simulink model "PC_Quadcopter_Simulation_Hexacopter_health_wind"  (R2022b)
settings: Solver=ode4  StartTime=0.0  StopTime=100  FixedStep=0.01  MaxStep=0.06  RelTol=1e-3
PreLoadFcn:
  | DoB_parameter
model workspace (MAT data in the model file):
  Sig : Simulink.Signal (value not decoded)
values from neighbouring files (symbols this model uses):
  A = [ ... (first row only)    [DoB_parameter.m]
  B = [0 1 0]'    [DoB_parameter.m]
  C = [1 0 0]    [DoB_parameter.m]
  den_Inv_X = conv(num_X,den_Qfilter)    [DoB_parameter.m]
  den_Inv_Y = conv(num_Y, den_Qfilter)    [DoB_parameter.m]
  den_Inv_Z = conv(num_Z, den_Qfilter_Z)    [DoB_parameter.m]
  den_Qfilter = [1 a1/tau a0/tau^2]    [DoB_parameter.m]
  den_Qfilter_Z = [1 a1/tau a0/tau^2]    [DoB_parameter.m]
  I_xx = J(1,1)    [DoB_parameter.m]
  I_yy = J(2,2)    [DoB_parameter.m]
  I_zz = J(3,3)    [DoB_parameter.m]
  IC = block.DialogPrm(2).Data    [quadcopterDynamicsSFunction.m]
  L = [l1 l2 l3]'    [DoB_parameter.m]
  num_Inv_X = conv(den_X,num_Qfilter)    [DoB_parameter.m]
  num_Inv_Y = conv(den_Y, num_Qfilter)    [DoB_parameter.m]
  num_Inv_Z = conv(den_Z, num_Qfilter_Z)    [DoB_parameter.m]
  num_Qfilter = a0/tau^2    (= 100)    [DoB_parameter.m]
  num_Qfilter_Z = a0/tau^2    (= 11.1111111111)    [DoB_parameter.m]
undefined symbols (not defined in the file or in its folder): F, Light, magnitude, MIL, quadModel
libraries: simulink x37, sharedTrackingLibrary x1, aerolibwind2 x1
(part 2 of 3)

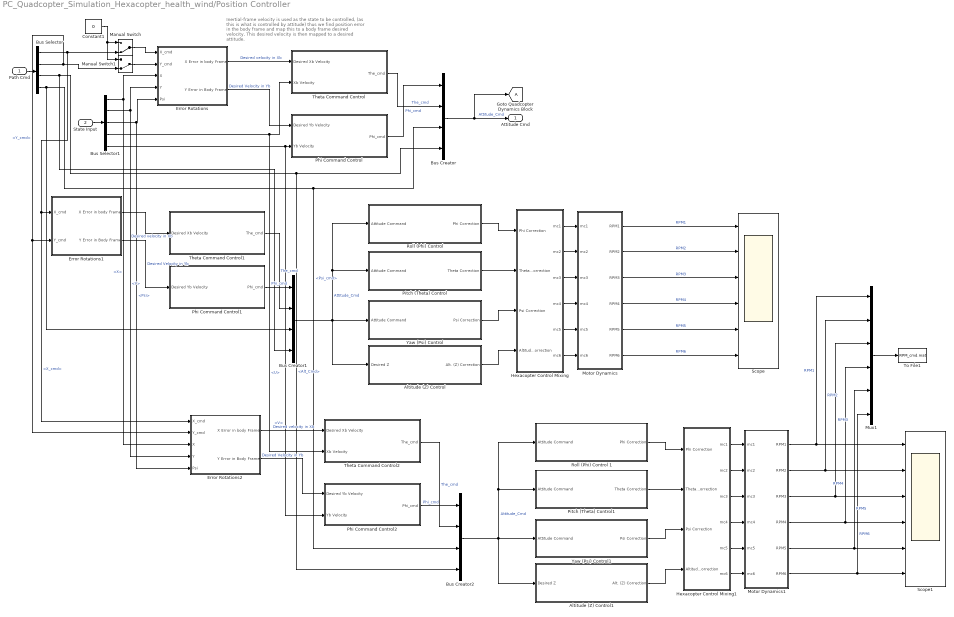
== system PC_Quadcopter_Simulation_Hexacopter_health_wind/Position Controller ==
  note: Inertial-frame velocity is used as the state to be controlled,
      | (as this is what is controlled by attitude)
      | thus we find position error in the body frame
      | and map this to a body frame desired velocity. This desired
      | velocity is then mapped to a desired attitude.
  Path Cmd : Inport
  State Input : Inport  Port=2
  Altitude (Z) Control : Subsystem  mask{Kpz=9, Kiz=6.6, Kdz=9.9, LimitOutput=on, USat=1, LSat=-1, GOffset=(sqrt((quadModel.mass*quadModel.g)/(6*quadModel.ct))-quadModel.b)/quadModel.cr}
      mask prompts: Kpz "Kp"; Kiz "Ki"; Kdz "Kd"; LimitOutput "Integral Saturation?"; USat "Upper saturation limit:"; LSat "Lower saturation limit:"; GOffset "Gravity Feedforward"
      mask help:
      | Adjust PID controller gains through this mask interface, or "look under mask" for more detailed adjustments.
      |
      | Note: Gravity Offset will not appear on block face as a value until simulation is run if it is the result of a formula involving the quadcopter model parameters.
      mask TypeOptions Kpz: Kpz/Gain
      mask TypeOptions Kiz: Kiz/Gain
      mask TypeOptions Kdz: Kdz/Gain
      mask TypeOptions LimitOutput:
      | Integrator
      | Limited/LimitOutput
      mask TypeOptions USat:
      | Integrator
      | Limited/UpperSaturationLimit
      mask TypeOptions LSat:
      | Integrator
      | Limited/LowerSaturationLimit
      mask TypeOptions GOffset: Gravity Offset (Level Flight)/Value
      mask Display:
      | fprintf(['Gravity Offset = ' num2str(GOffset) '\n' ...
      |     'Kp = ' num2str(Kpz) '\n' ...
      |     'Ki = ' num2str(Kiz) '\n' ...
      |     'Kd = ' num2str(Kdz) '\n' ...
      |     'Integral Saturation: ' LimitOutput]);
      | if strcmp(LimitOutput,'on')
      |     fprintf([' \n' ' \n' ' \n' ' \n' ' \n' '\n' ...
      |         'Limits: ' num2str(USat) ' to ' num2str(LSat)]);
      | end
  Altitude (Z) Control1 : Subsystem  mask{Kpz=9, Kiz=6.6, Kdz=9.9, LimitOutput=on, USat=1, LSat=-1, GOffset=(sqrt((quadModel.mass*quadModel.g)/(6*quadModel.ct))-quadModel.b)/quadModel.cr}
      mask prompts: Kpz "Kp"; Kiz "Ki"; Kdz "Kd"; LimitOutput "Integral Saturation?"; USat "Upper saturation limit:"; LSat "Lower saturation limit:"; GOffset "Gravity Feedforward"
      mask help:
      | Adjust PID controller gains through this mask interface, or "look under mask" for more detailed adjustments.
      |
      | Note: Gravity Offset will not appear on block face as a value until simulation is run if it is the result of a formula involving the quadcopter model parameters.
      mask TypeOptions Kpz: Kpz/Gain
      mask TypeOptions Kiz: Kiz/Gain
      mask TypeOptions Kdz: Kdz/Gain
      mask TypeOptions LimitOutput:
      | Integrator
      | Limited/LimitOutput
      mask TypeOptions USat:
      | Integrator
      | Limited/UpperSaturationLimit
      mask TypeOptions LSat:
      | Integrator
      | Limited/LowerSaturationLimit
      mask TypeOptions GOffset: Gravity Offset (Level Flight)/Value
      mask Display:
      | fprintf(['Gravity Offset = ' num2str(GOffset) '\n' ...
      |     'Kp = ' num2str(Kpz) '\n' ...
      |     'Ki = ' num2str(Kiz) '\n' ...
      |     'Kd = ' num2str(Kdz) '\n' ...
      |     'Integral Saturation: ' LimitOutput]);
      | if strcmp(LimitOutput,'on')
      |     fprintf([' \n' ' \n' ' \n' ' \n' ' \n' '\n' ...
      |         'Limits: ' num2str(USat) ' to ' num2str(LSat)]);
      | end
  Bus Creator : BusCreator  Inputs=4
  Bus Creator1 : BusCreator  Inputs=4
  Bus Creator2 : BusCreator  Inputs=4
  Bus Selector : BusSelector  OutputSignals=X_cmd,Y_cmd,Alt_Cmd,Psi_cmd
  Bus Selector1 : BusSelector  OutputSignals=X,Y,Psi,U,V
  Constant1 : Constant  Value=0
  Error Rotations : Subsystem
  Error Rotations1 : Subsystem
  Error Rotations2 : Subsystem
  Goto Quadcopter Dynamics Block : Goto  TagVisibility=global
  Hexacopter Control Mixing : Subsystem
      mask Display:
      | modelLoaded = evalin('base','exist(''quadModel'',''var'')');
      | if (modelLoaded==1)
      |     if (evalin('base','quadModel.plusConfig'))
      |     fprintf([' \n' ' \n'  'Configuration "+"']);
      |     else if (~evalin('base','quadModel.plusConfig'))
      |         fprintf([' \n' ' \n' 'Configuration "X"']);
      |         end
      |     end
      | else
      |     fprintf([' \n' ' \n'  'Model Not Loaded']);
      | end
  Hexacopter Control Mixing1 : Subsystem
      mask Display:
      | modelLoaded = evalin('base','exist(''quadModel'',''var'')');
      | if (modelLoaded==1)
      |     if (evalin('base','quadModel.plusConfig'))
      |     fprintf([' \n' ' \n'  'Configuration "+"']);
      |     else if (~evalin('base','quadModel.plusConfig'))
      |         fprintf([' \n' ' \n' 'Configuration "X"']);
      |         end
      |     end
      | else
      |     fprintf([' \n' ' \n'  'Model Not Loaded']);
      | end
  Manual Switch : ManualSwitch  CurrentSetting=0
  Manual Switch1 : ManualSwitch  CurrentSetting=0
  Motor Dynamics : Subsystem
  Motor Dynamics1 : Subsystem
  Mux1 : Mux  Inputs=6
  Phi Command Control : Subsystem  mask{Kp=0.32, Kd=0.1, ASat=20*pi/180}
      mask prompts: Kp "Proportional Gain"; Kd "Derivative Gain"; ASat "Attitude Limit (+/- radians):"
      mask TypeOptions Kp: Kpp/Gain
      mask TypeOptions Kd: Kdp/Gain
      mask TypeOptions ASat: Attitude Limits_Phi/UpperLimit
      mask Display:
      | fprintf(['Kp = ' num2str(Kp) '\n' ...
      |     'Kd = ' num2str(Kd) '\n' ...
      |     'Attitude Limit (+/-): ' num2str(ASat*180/pi) '°']);
  Phi Command Control1 : Subsystem  mask{Kp=0.32, Kd=0.1, ASat=20*pi/180}
      mask prompts: Kp "Proportional Gain"; Kd "Derivative Gain"; ASat "Attitude Limit (+/- radians):"
      mask TypeOptions Kp: Kpp/Gain
      mask TypeOptions Kd: Kdp/Gain
      mask TypeOptions ASat: Attitude Limits_Phi/UpperLimit
      mask Display:
      | fprintf(['Kp = ' num2str(Kp) '\n' ...
      |     'Kd = ' num2str(Kd) '\n' ...
      |     'Attitude Limit (+/-): ' num2str(ASat*180/pi) '°']);
  Phi Command Control2 : Subsystem  mask{Kp=0.32, Kd=0.1, ASat=20*pi/180}
      mask prompts: Kp "Proportional Gain"; Kd "Derivative Gain"; ASat "Attitude Limit (+/- radians):"
      mask TypeOptions Kp: Kpp/Gain
      mask TypeOptions Kd: Kdp/Gain
      mask TypeOptions ASat: Attitude Limits_Phi/UpperLimit
      mask Display:
      | fprintf(['Kp = ' num2str(Kp) '\n' ...
      |     'Kd = ' num2str(Kd) '\n' ...
      |     'Attitude Limit (+/-): ' num2str(ASat*180/pi) '°']);
  Pitch (Theta) Control : Subsystem  mask{Kpt=2, Kit=1.1, Kdt=1.2, LimitOutput=on, USat=1, LSat=-1}
      mask prompts: Kpt "Kp"; Kit "Ki"; Kdt "Kd"; LimitOutput "Integral Saturation?"; USat "Upper saturation limit:"; LSat "Lower saturation limit:"
      mask help: Adjust PID controller gains through this mask interface, or "look under mask" for more detailed adjustments.
      mask TypeOptions Kpt: Kpt/Gain
      mask TypeOptions Kit: Kit/Gain
      mask TypeOptions Kdt: Kdt/Gain
      mask TypeOptions LimitOutput:
      | Integrator
      | Limited/LimitOutput
      mask TypeOptions USat:
      | Integrator
      | Limited/UpperSaturationLimit
      mask TypeOptions LSat:
      | Integrator
      | Limited/LowerSaturationLimit
      mask Display:
      | fprintf(['Kp = ' num2str(Kpt) '\n' ...
      |     'Ki = ' num2str(Kit) '\n' ...
      |     'Kd = ' num2str(Kdt) '\n' ...
      |     'Integral Saturation: ' LimitOutput]);
      | if strcmp(LimitOutput,'on')
      |     fprintf([' \n' ' \n' ' \n' ' \n' '\n' ...
      |         'Limits: ' num2str(USat) ' to ' num2str(LSat)]);
      | end
  Pitch (Theta) Control1 : Subsystem  mask{Kpt=2, Kit=1.1, Kdt=1.2, LimitOutput=on, USat=1, LSat=-1}
      mask prompts: Kpt "Kp"; Kit "Ki"; Kdt "Kd"; LimitOutput "Integral Saturation?"; USat "Upper saturation limit:"; LSat "Lower saturation limit:"
      mask help: Adjust PID controller gains through this mask interface, or "look under mask" for more detailed adjustments.
      mask TypeOptions Kpt: Kpt/Gain
      mask TypeOptions Kit: Kit/Gain
      mask TypeOptions Kdt: Kdt/Gain
      mask TypeOptions LimitOutput:
      | Integrator
      | Limited/LimitOutput
      mask TypeOptions USat:
      | Integrator
      | Limited/UpperSaturationLimit
      mask TypeOptions LSat:
      | Integrator
      | Limited/LowerSaturationLimit
      mask Display:
      | fprintf(['Kp = ' num2str(Kpt) '\n' ...
      |     'Ki = ' num2str(Kit) '\n' ...
      |     'Kd = ' num2str(Kdt) '\n' ...
      |     'Integral Saturation: ' LimitOutput]);
      | if strcmp(LimitOutput,'on')
      |     fprintf([' \n' ' \n' ' \n' ' \n' '\n' ...
      |         'Limits: ' num2str(USat) ' to ' num2str(LSat)]);
      | end
  "Roll (Phi) Control " : Subsystem  mask{Kpp=2, Kip=1.1, Kdp=1.2, LimitOutput=on, USat=1, LSat=-1}
      mask prompts: Kpp "Kp"; Kip "Ki"; Kdp "Kd"; LimitOutput "Integral Saturation:"; USat "Upper saturation limit:"; LSat "Lower saturation limit:"
      mask help:
      | Adjust PID controller gains through this mask interface, or "look under mask"
      | for more detailed adjustments.
      mask TypeOptions Kpp: Kpp/Gain
      mask TypeOptions Kip: Kip/Gain
      mask TypeOptions Kdp: Kdp/Gain
      mask TypeOptions LimitOutput:
      | Integrator
      | Limited/LimitOutput
      mask TypeOptions USat:
      | Integrator
      | Limited/UpperSaturationLimit
      mask TypeOptions LSat:
      | Integrator
      | Limited/LowerSaturationLimit
      mask Display:
      | fprintf(['Kp = ' num2str(Kpp) '\n' ...
      |     'Ki = ' num2str(Kip) '\n' ...
      |     'Kd = ' num2str(Kdp) '\n'...
      |     'Integral Saturation: ' LimitOutput]);
      | if strcmp(LimitOutput,'on')
      |     fprintf([' \n' ' \n' ' \n' ' \n' '\n' ...
      |         'Limits: ' num2str(USat) ' to ' num2str(LSat)]);
      | end
  Roll (Phi) Control 1 : Subsystem  mask{Kpp=2, Kip=1.1, Kdp=1.2, LimitOutput=on, USat=1, LSat=-1}
      mask prompts: Kpp "Kp"; Kip "Ki"; Kdp "Kd"; LimitOutput "Integral Saturation:"; USat "Upper saturation limit:"; LSat "Lower saturation limit:"
      mask help:
      | Adjust PID controller gains through this mask interface, or "look under mask"
      | for more detailed adjustments.
      mask TypeOptions Kpp: Kpp/Gain
      mask TypeOptions Kip: Kip/Gain
      mask TypeOptions Kdp: Kdp/Gain
      mask TypeOptions LimitOutput:
      | Integrator
      | Limited/LimitOutput
      mask TypeOptions USat:
      | Integrator
      | Limited/UpperSaturationLimit
      mask TypeOptions LSat:
      | Integrator
      | Limited/LowerSaturationLimit
      mask Display:
      | fprintf(['Kp = ' num2str(Kpp) '\n' ...
      |     'Ki = ' num2str(Kip) '\n' ...
      |     'Kd = ' num2str(Kdp) '\n'...
      |     'Integral Saturation: ' LimitOutput]);
      | if strcmp(LimitOutput,'on')
      |     fprintf([' \n' ' \n' ' \n' ' \n' '\n' ...
      |         'Limits: ' num2str(USat) ' to ' num2str(LSat)]);
      | end
  Scope : Scope  NumInputPorts=6
  Scope1 : Scope  NumInputPorts=6
  Theta Command Control : Subsystem  mask{Kp=0.32, Kd=0.1, ASat=20*pi/180}
      mask prompts: Kp "Proportional Gain:"; Kd "Derivative Gain"; ASat "Attitude Limit (+/- radians):"
      mask TypeOptions Kp: Kpt/Gain
      mask TypeOptions Kd: Kdt/Gain
      mask TypeOptions ASat: Attitude Limits_Theta/UpperLimit
      mask Display:
      | fprintf(['Kp = ' num2str(Kp) '\n' ...
      |     'Kd = ' num2str(Kd) '\n' ...
      |     'Attitude Limit (+/-): ' num2str(ASat*180/pi) '°']);
  Theta Command Control1 : Subsystem  mask{Kp=0.32, Kd=0.1, ASat=20*pi/180}
      mask prompts: Kp "Proportional Gain:"; Kd "Derivative Gain"; ASat "Attitude Limit (+/- radians):"
      mask TypeOptions Kp: Kpt/Gain
      mask TypeOptions Kd: Kdt/Gain
      mask TypeOptions ASat: Attitude Limits_Theta/UpperLimit
      mask Display:
      | fprintf(['Kp = ' num2str(Kp) '\n' ...
      |     'Kd = ' num2str(Kd) '\n' ...
      |     'Attitude Limit (+/-): ' num2str(ASat*180/pi) '°']);
  Theta Command Control2 : Subsystem  mask{Kp=0.32, Kd=0.1, ASat=20*pi/180}
      mask prompts: Kp "Proportional Gain:"; Kd "Derivative Gain"; ASat "Attitude Limit (+/- radians):"
      mask TypeOptions Kp: Kpt/Gain
      mask TypeOptions Kd: Kdt/Gain
      mask TypeOptions ASat: Attitude Limits_Theta/UpperLimit
      mask Display:
      | fprintf(['Kp = ' num2str(Kp) '\n' ...
      |     'Kd = ' num2str(Kd) '\n' ...
      |     'Attitude Limit (+/-): ' num2str(ASat*180/pi) '°']);
  To File1 : ToFile  Filename=RPM_cmd.mat  MatrixName=RPM_cmd  SaveFormat=Timeseries
  Yaw (Psi) Control : Subsystem  mask{Kps=0.3, Kis=0.15, Kds=0.5, LimitOutput=on, USat=1, LSat=-1}
      mask prompts: Kps "Kp"; Kis "Ki"; Kds "Kd"; LimitOutput "Integral Saturation?"; USat "Upper saturation limit:"; LSat "Lower saturation limit:"
      mask help: Adjust PID controller gains through this mask interface, or "look under mask" for more detailed adjustments.
      mask TypeOptions Kps: Kps/Gain
      mask TypeOptions Kis: Kit/Gain
      mask TypeOptions Kds: Kds/Gain
      mask TypeOptions LimitOutput:
      | Integrator
      | Limited/LimitOutput
      mask TypeOptions USat:
      | Integrator
      | Limited/UpperSaturationLimit
      mask TypeOptions LSat:
      | Integrator
      | Limited/LowerSaturationLimit
      mask Display:
      | fprintf(['Kp = ' num2str(Kps) '\n' ...
      |     'Ki = ' num2str(Kis) '\n' ...
      |     'Kd = ' num2str(Kds) '\n' ...
      |     'Integral Saturation: ' LimitOutput]);
      | if strcmp(LimitOutput,'on')
      |     fprintf([' \n' ' \n' ' \n' ' \n' '\n' ...
      |         'Limits: ' num2str(USat) ' to ' num2str(LSat)]);
      | end
  Yaw (Psi) Control1 : Subsystem  mask{Kps=0.3, Kis=0.15, Kds=0.5, LimitOutput=on, USat=1, LSat=-1}
      mask prompts: Kps "Kp"; Kis "Ki"; Kds "Kd"; LimitOutput "Integral Saturation?"; USat "Upper saturation limit:"; LSat "Lower saturation limit:"
      mask help: Adjust PID controller gains through this mask interface, or "look under mask" for more detailed adjustments.
      mask TypeOptions Kps: Kps/Gain
      mask TypeOptions Kis: Kit/Gain
      mask TypeOptions Kds: Kds/Gain
      mask TypeOptions LimitOutput:
      | Integrator
      | Limited/LimitOutput
      mask TypeOptions USat:
      | Integrator
      | Limited/UpperSaturationLimit
      mask TypeOptions LSat:
      | Integrator
      | Limited/LowerSaturationLimit
      mask Display:
      | fprintf(['Kp = ' num2str(Kps) '\n' ...
      |     'Ki = ' num2str(Kis) '\n' ...
      |     'Kd = ' num2str(Kds) '\n' ...
      |     'Integral Saturation: ' LimitOutput]);
      | if strcmp(LimitOutput,'on')
      |     fprintf([' \n' ' \n' ' \n' ' \n' '\n' ...
      |         'Limits: ' num2str(USat) ' to ' num2str(LSat)]);
      | end
  Attitude Cmd : Outport
  wires:
  Motor Dynamics/6(RPM6) -> Scope/6  "RPM6"
  Manual Switch/1 -> Error Rotations/1(X_cmd)
  Phi Command Control1/1(Phi_cmd) -> Bus Creator1/1  "Phi_cmd"
  Hexacopter Control Mixing/1(mc1) -> Motor Dynamics/1(mc1)
  Yaw (Psi) Control/1(Psi Correction) -> Hexacopter Control Mixing/3(Psi Correction)
  Motor Dynamics/5(RPM5) -> Scope/5  "RPM5"
  Hexacopter Control Mixing/6(mc6) -> Motor Dynamics/6(mc6)
  Theta Command Control1/1(The_cmd) -> Bus Creator1/2  "The_cmd"
  Bus Creator/1 -> Attitude Cmd/1, Goto Quadcopter Dynamics Block/1  "Attitude_Cmd"
  Bus Selector/1 -> Error Rotations2/1(X_cmd), Error Rotations1/1(X_cmd), Manual Switch/2  "<X_cmd>"
  Motor Dynamics/2(RPM2) -> Scope/2  "RPM2"
  Altitude (Z) Control/1(Alt. (Z) Correction) -> Hexacopter Control Mixing/4(Altitude Correction)
  Motor Dynamics/3(RPM3) -> Scope/3  "RPM3"
  Constant1/1 -> Manual Switch1/1, Manual Switch/1
  Bus Creator1/1 -> Pitch (Theta) Control/1(Attitude Command), "Roll (Phi) Control "/1("Attitude Command "), Yaw (Psi) Control/1(Attitude Command), Altitude (Z) Control/1(Desired Z)  "Attitude_Cmd"
  Error Rotations/2(Y Error in Body Frame) -> Phi Command Control/1(Desired Yb Velocity)  "Desired Velocity in Yb"
  Bus Selector/3 -> Bus Creator1/4, Bus Creator2/4, Bus Creator/4  "<Alt_Cmd>"
  "Roll (Phi) Control "/1(Phi Correction) -> Hexacopter Control Mixing/1(Phi Correction)
  Bus Selector/2 -> Error Rotations2/2(Y_cmd), Error Rotations1/2(Y_cmd), Manual Switch1/2  "<Y_cmd>"
  Error Rotations1/2(Y Error in Body Frame) -> Phi Command Control1/1(Desired Yb Velocity)  "Desired Velocity in Yb"
  Path Cmd/1 -> Bus Selector/1
  Hexacopter Control Mixing/4(mc4) -> Motor Dynamics/4(mc4)
  Phi Command Control/1(Phi_cmd) -> Bus Creator/1  "Phi_cmd"
  Motor Dynamics/1(RPM1) -> Scope/1  "RPM1"
  Pitch (Theta) Control/1(Theta Correction) -> Hexacopter Control Mixing/2(Theta Correction)
  Error Rotations/1(X Error in body Frame) -> Theta Command Control/1(Desired Xb Velocity)  "Desired velocity in Xb"
  Error Rotations1/1(X Error in body Frame) -> Theta Command Control1/1(Desired Xb Velocity)  "Desired velocity in Xb"
  Hexacopter Control Mixing/5(mc5) -> Motor Dynamics/5(mc5)
  Manual Switch1/1 -> Error Rotations/2(Y_cmd)
  Hexacopter Control Mixing/3(mc3) -> Motor Dynamics/3(mc3)
  Theta Command Control/1(The_cmd) -> Bus Creator/2  "The_cmd"
  Hexacopter Control Mixing/2(mc2) -> Motor Dynamics/2(mc2)
  State Input/1 -> Bus Selector1/1
  Bus Selector/4 -> Bus Creator1/3, Bus Creator2/3, Bus Creator/3  "<Psi_cmd>"
  Motor Dynamics/4(RPM4) -> Scope/4  "RPM4"
  Motor Dynamics1/4(RPM4) -> Mux1/4, Scope1/4  "RPM4"
  Hexacopter Control Mixing1/2(mc2) -> Motor Dynamics1/2(mc2)
  Hexacopter Control Mixing1/3(mc3) -> Motor Dynamics1/3(mc3)
  Hexacopter Control Mixing1/5(mc5) -> Motor Dynamics1/5(mc5)
  Pitch (Theta) Control1/1(Theta Correction) -> Hexacopter Control Mixing1/2(Theta Correction)
  Motor Dynamics1/1(RPM1) -> Mux1/1, Scope1/1  "RPM1"
  Hexacopter Control Mixing1/4(mc4) -> Motor Dynamics1/4(mc4)
  Roll (Phi) Control 1/1(Phi Correction) -> Hexacopter Control Mixing1/1(Phi Correction)
  Bus Creator2/1 -> Altitude (Z) Control1/1(Desired Z), Yaw (Psi) Control1/1(Attitude Command), Roll (Phi) Control 1/1("Attitude Command "), Pitch (Theta) Control1/1(Attitude Command)  "Attitude_Cmd"
  Motor Dynamics1/3(RPM3) -> Mux1/3, Scope1/3  "RPM3"
  Altitude (Z) Control1/1(Alt. (Z) Correction) -> Hexacopter Control Mixing1/4(Altitude Correction)
  Motor Dynamics1/2(RPM2) -> Mux1/2, Scope1/2  "RPM2"
  Hexacopter Control Mixing1/6(mc6) -> Motor Dynamics1/6(mc6)
  Motor Dynamics1/5(RPM5) -> Mux1/5, Scope1/5  "RPM5"
  Yaw (Psi) Control1/1(Psi Correction) -> Hexacopter Control Mixing1/3(Psi Correction)
  Hexacopter Control Mixing1/1(mc1) -> Motor Dynamics1/1(mc1)
  Motor Dynamics1/6(RPM6) -> Mux1/6, Scope1/6  "RPM6"
  Bus Selector1/2 -> Error Rotations2/4(Y), Error Rotations/4(Y)  "<Y>"
  Bus Selector1/5 -> Phi Command Control2/2(Yb Velocity), Phi Command Control/2(Yb Velocity)  "<V>"
  Bus Selector1/3 -> Error Rotations2/5(Psi), Error Rotations/5(Psi)  "<Psi>"
  Bus Selector1/1 -> Error Rotations/3(X), Error Rotations2/3(X)  "<X>"
  Error Rotations2/1(X Error in body Frame) -> Theta Command Control2/1(Desired Xb Velocity)  "Desired velocity in Xb"
  Error Rotations2/2(Y Error in Body Frame) -> Phi Command Control2/1(Desired Yb Velocity)  "Desired Velocity in Yb"
  Bus Selector1/4 -> Theta Command Control2/2(Xb Velocity), Theta Command Control/2(Xb Velocity)  "<U>"
  Theta Command Control2/1(The_cmd) -> Bus Creator2/2  "The_cmd"
  Phi Command Control2/1(Phi_cmd) -> Bus Creator2/1  "Phi_cmd"
  Mux1/1 -> To File1/1

== system PC_Quadcopter_Simulation_Hexacopter_health_wind/Attitude Controller/Altitude (Z) Control ==
  note: Improve to use rotation matrix and euler angles...
      | maybe with saturation?
  note: ez
  Desired Z : Inport
  Z State : Inport  Port=2
  Bus Selector : BusSelector  OutputSignals=Alt_Cmd
  Derivative : Derivative
  Gravity Offset (Level Flight) : Constant  Value=GOffset
  Integrator Limited : Integrator  LimitOutput=on  UpperSaturationLimit=USat  LowerSaturationLimit=LSat
  Kdz : Gain  Gain=Kdz
  Kiz : Gain  Gain=Kiz
  Kpz : Gain  Gain=Kpz
  Sum : Sum  Inputs=|+-
  Sum2 : Sum  Inputs=+++-
  Alt. (Z) Correction : Outport
  wires:
  Gravity Offset (Level Flight)/1 -> Sum2/1
  Desired Z/1 -> Bus Selector/1
  Z State/1 -> Derivative/1, Sum/2
  Sum2/1 -> Alt. (Z) Correction/1
  Kpz/1 -> Sum2/2  "P Corr"
  Sum/1 -> Integrator Limited/1, Kpz/1  "Error"
  Kiz/1 -> Sum2/3  "I Corr"
  Kdz/1 -> Sum2/4  "D Corr"
  Integrator Limited/1 -> Kiz/1
  Bus Selector/1 -> Sum/1  "<Alt_Cmd>"
  Derivative/1 -> Kdz/1

== system PC_Quadcopter_Simulation_Hexacopter_health_wind/Attitude Controller/Pitch (Theta) Control ==
  Attitude Command : Inport
  Theta State : Inport  Port=2
  P State : Inport  Port=3
  Bus Selector : BusSelector  OutputSignals=The_cmd
  Integrator Limited : Integrator  LimitOutput=on  UpperSaturationLimit=USat  LowerSaturationLimit=LSat
  Kdt : Gain  Gain=Kdt
  Kit : Gain  Gain=Kit
  Kpt : Gain  Gain=Kpt
  Sum : Sum  Inputs=|+-
  Sum1 : Sum  Inputs=++-
  Theta Correction : Outport
  wires:
  Sum/1 -> Integrator Limited/1, Kpt/1  "Error"
  Attitude Command/1 -> Bus Selector/1
  Theta State/1 -> Sum/2
  Sum1/1 -> Theta Correction/1
  Kpt/1 -> Sum1/1  "P Corr"
  Kdt/1 -> Sum1/3  "D Corr"
  Kit/1 -> Sum1/2  "I Corr"
  Integrator Limited/1 -> Kit/1
  Bus Selector/1 -> Sum/1  "<The_cmd>"
  P State/1 -> Kdt/1

== system PC_Quadcopter_Simulation_Hexacopter_health_wind/Attitude Controller/Roll (Phi) Control  ==
  "Attitude Command " : Inport
  Phi State : Inport  Port=2
  P : Inport  Port=3
  Bus Selector : BusSelector  OutputSignals=Phi_cmd
  Integrator Limited : Integrator  LimitOutput=on  UpperSaturationLimit=USat  LowerSaturationLimit=LSat
  Kdp : Gain  Gain=Kdp
  Kip : Gain  Gain=Kip
  Kpp : Gain  Gain=Kpp
  Sum : Sum  Inputs=|+-
  Sum1 : Sum  Inputs=++-
  Phi Correction : Outport
  wires:
  Sum/1 -> Integrator Limited/1, Kpp/1  "Error"
  Phi State/1 -> Sum/2
  Sum1/1 -> Phi Correction/1
  Kpp/1 -> Sum1/1  "P Corr"
  Kdp/1 -> Sum1/3  "D Corr"
  Kip/1 -> Sum1/2  "I Corr"
  Integrator Limited/1 -> Kip/1
  "Attitude Command "/1 -> Bus Selector/1
  Bus Selector/1 -> Sum/1  "<Phi_cmd>"
  P/1 -> Kdp/1

== system PC_Quadcopter_Simulation_Hexacopter_health_wind/Attitude Controller/Yaw (Psi) Control ==
  Attitude Command : Inport
  Psi State : Inport  Port=2
  R State : Inport  Port=3
  Bus Selector : BusSelector  OutputSignals=Psi_cmd
  Integrator Limited : Integrator  LimitOutput=on  UpperSaturationLimit=USat  LowerSaturationLimit=LSat
  Kds : Gain  Gain=Kds
  Kit : Gain  Gain=Kis
  Kps : Gain  Gain=Kps
  Sum : Sum  Inputs=|+-
  Sum1 : Sum  Inputs=++-
  Psi Correction : Outport
  wires:
  Sum/1 -> Integrator Limited/1, Kps/1  "Error"
  Attitude Command/1 -> Bus Selector/1
  Sum1/1 -> Psi Correction/1
  Psi State/1 -> Sum/2
  Kps/1 -> Sum1/1  "P Corr"
  Kds/1 -> Sum1/3  "D Corr"
  Kit/1 -> Sum1/2  "I Corr"
  Integrator Limited/1 -> Kit/1
  Bus Selector/1 -> Sum/1  "<Psi_cmd>"
  R State/1 -> Kds/1

== system PC_Quadcopter_Simulation_Hexacopter_health_wind/DOB/Subsystem ==
  PID_X : Inport
  Angle_X : Inport  Port=2
  Sum : Sum  Inputs=|-+
  Transfer Fcn : TransferFcn  Numerator=num_Qfilter  Denominator=den_Qfilter
  Transfer Fcn1 : TransferFcn  Numerator=num_Inv_X  Denominator=den_Inv_X
  DOB_X : Outport
  wires:
  PID_X/1 -> Transfer Fcn/1
  Transfer Fcn/1 -> Sum/1
  Transfer Fcn1/1 -> Sum/2
  Angle_X/1 -> Transfer Fcn1/1
  Sum/1 -> DOB_X/1

== system PC_Quadcopter_Simulation_Hexacopter_health_wind/DOB/Subsystem1 ==
  PID_Y : Inport
  Anlgel_Y : Inport  Port=2
  Sum : Sum  Inputs=|-+
  Transfer Fcn : TransferFcn  Numerator=num_Qfilter  Denominator=den_Qfilter
  Transfer Fcn1 : TransferFcn  Numerator=num_Inv_Y  Denominator=den_Inv_Y
  DOB_Y : Outport
  wires:
  PID_Y/1 -> Transfer Fcn/1
  Transfer Fcn/1 -> Sum/1
  Transfer Fcn1/1 -> Sum/2
  Anlgel_Y/1 -> Transfer Fcn1/1
  Sum/1 -> DOB_Y/1

== system PC_Quadcopter_Simulation_Hexacopter_health_wind/DOB/Subsystem2 ==
  PID_Z : Inport
  Angle_Z : Inport  Port=2
  Q filter A : TransferFcn  Numerator=num_Qfilter_Z  Denominator=den_Qfilter_Z
  Q filter B + Pn^-1(s) : TransferFcn  Numerator=num_Inv_Z  Denominator=den_Inv_Z
  Sum : Sum  Inputs=|-+
  DOB_Z : Outport
  wires:
  PID_Z/1 -> Q filter A/1
  Q filter A/1 -> Sum/1
  Q filter B + Pn^-1(s)/1 -> Sum/2
  Angle_Z/1 -> Q filter B + Pn^-1(s)/1
  Sum/1 -> DOB_Z/1

== system PC_Quadcopter_Simulation_Hexacopter_health_wind/Fault Diagnosis/Generate Residual ==
  yMeasured[k] : Inport
  xEstimated[k|k] : Inport  Port=2
  RPM command : Inport  Port=3
  MATLAB Function - Generate Predicted Output : MATLAB Function  TreatAsAtomicUnit=on
  Subtract : Sum  Inputs=+-
  Unit Delay : UnitDelay  InitialCondition=zeros(15,1)  SampleTime=-1  HasFrameUpgradeWarning=on
  Residual : Outport
  wires:
  xEstimated[k|k]/1 -> Unit Delay/1
  Unit Delay/1 -> MATLAB Function - Generate Predicted Output/1(xEstimated)  "xEstimated[k-1|k-1]"
  MATLAB Function - Generate Predicted Output/1(yPredicted) -> Subtract/2  "yPredicted[k|k-1]"
  Subtract/1 -> Residual/1  "e[k]"
  yMeasured[k]/1 -> Subtract/1
  RPM command/1 -> MATLAB Function - Generate Predicted Output/2(u)

== system PC_Quadcopter_Simulation_Hexacopter_health_wind/Hexacopter Dynamics/External Disturbances ==
  note: Note: Torques are in units of N*m, Forces in N
      | Torques are applied to the BODY coordinate system.
      | Forces are applied from the WORLD coordinate system!
      | This can be changed by adjusting the equations within the S-function.
  Bus Creator : BusCreator  Inputs=6
  Bus to Vector : BusToVector
  Constant{1..2,5..6} (4 alike) : Constant  Value=0
  Manual Switch : ManualSwitch
  Manual Switch1 : ManualSwitch
  Step : Step  Time=5  After=0.1  SampleTime=0
  Step2 : Step  Time=10  After=3  SampleTime=0
  "Disturbances " : Outport
  wires:
  Bus to Vector/1 -> "Disturbances "/1
  Bus Creator/1 -> Bus to Vector/1
  Constant6/1 -> Manual Switch1/1, Bus Creator/1  "Tau_bx-axis"
  Constant2/1 -> Bus Creator/3  "Tau_bz-axis"
  Constant1/1 -> Manual Switch/1, Bus Creator/4  "Force_x-axis"
  Constant5/1 -> Bus Creator/6  "Force_z-axis"
  Manual Switch/1 -> Bus Creator/5
  Step2/1 -> Manual Switch/2  "Force_y-axis"
  Manual Switch1/1 -> Bus Creator/2
  Step/1 -> Manual Switch1/2  "Tau_by-axis"

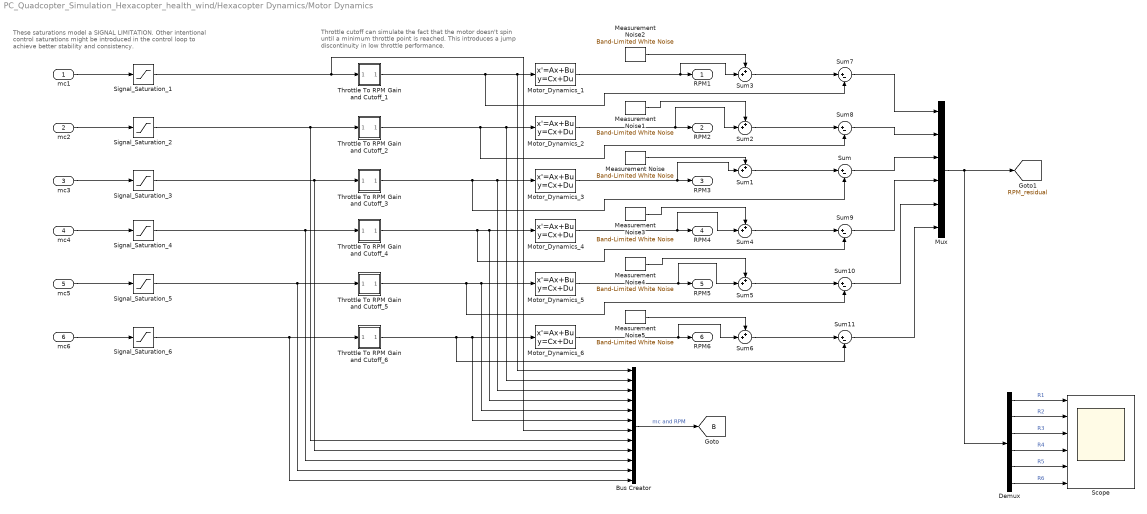
== system PC_Quadcopter_Simulation_Hexacopter_health_wind/Hexacopter Dynamics/Motor Dynamics ==
  note: Throttle cutoff can simulate the fact that the motor doesn't
      | spin until a minimum throttle point is reached. This introduces
      | a jump discontinuity in low throttle performance.
  note: These saturations model a SIGNAL LIMITATION.
      | Other intentional control saturations might be introduced in the
      | control loop to achieve better stability and consistency.
  mc1 : Inport
  mc2 : Inport  Port=2
  mc3 : Inport  Port=3
  mc4 : Inport  Port=4
  mc5 : Inport  Port=5
  mc6 : Inport  Port=6
  Bus Creator : BusCreator  Inputs=12
  Demux : Demux  Outputs=6
  Measurement Noise{,1..5} (6 alike) : simulink/Sources/Band-Limited White Noise  Cov=10^2  Ts=0.02  seed=[23342]
  Motor_Dynamics_1 : StateSpace  A=-1/quadModel.T  C=1/quadModel.T  D=0  InitialCondition=IC.w1*quadModel.T
  Motor_Dynamics_2 : StateSpace  A=-1/quadModel.T  C=1/quadModel.T  D=0  InitialCondition=IC.w2*quadModel.T
  Motor_Dynamics_3 : StateSpace  A=-1/quadModel.T  C=1/quadModel.T  D=0  InitialCondition=IC.w3*quadModel.T
  Motor_Dynamics_4 : StateSpace  A=-1/quadModel.T  C=1/quadModel.T  D=0  InitialCondition=IC.w4*quadModel.T
  Motor_Dynamics_5 : StateSpace  A=-1/quadModel.T  C=1/quadModel.T  D=0  InitialCondition=IC.w4*quadModel.T
  Motor_Dynamics_6 : StateSpace  A=-1/quadModel.T  C=1/quadModel.T  D=0  InitialCondition=IC.w4*quadModel.T
  Mux : Mux  Inputs=6
  Scope : Scope  NumInputPorts=6
  Signal_Saturation_{1..6} (6 alike) : Saturate  UpperLimit=100  LowerLimit=0
  Sum{,7..11} (6 alike) : Sum  Inputs=|+-
  Sum{1..6} (6 alike) : Sum  Inputs=++|
  Throttle To RPM Gain and Cutoff_1 : Subsystem
  Throttle To RPM Gain and Cutoff_2 : Subsystem
  Throttle To RPM Gain and Cutoff_3 : Subsystem
  Throttle To RPM Gain and Cutoff_4 : Subsystem
  Throttle To RPM Gain and Cutoff_5 : Subsystem
  Throttle To RPM Gain and Cutoff_6 : Subsystem
  RPM1 : Outport
  RPM2 : Outport  Port=2
  RPM3 : Outport  Port=3
  RPM4 : Outport  Port=4
  RPM5 : Outport  Port=5
  RPM6 : Outport  Port=6
  tag scope: B=global, RPM_residual=global
  wires:
  mc1/1 -> Signal_Saturation_1/1
  mc4/1 -> Signal_Saturation_4/1
  mc2/1 -> Signal_Saturation_2/1
  mc3/1 -> Signal_Saturation_3/1
  Signal_Saturation_1/1 -> Bus Creator/7, Throttle To RPM Gain and Cutoff_1/1(In5)
  Signal_Saturation_2/1 -> Throttle To RPM Gain and Cutoff_2/1(In5), Bus Creator/8
  Signal_Saturation_3/1 -> Bus Creator/9, Throttle To RPM Gain and Cutoff_3/1(In5)
  Signal_Saturation_4/1 -> Bus Creator/10, Throttle To RPM Gain and Cutoff_4/1(In5)
  Throttle To RPM Gain and Cutoff_1/1(Out5) -> Sum7/2, Bus Creator/1, Motor_Dynamics_1/1
  Throttle To RPM Gain and Cutoff_2/1(Out5) -> Sum8/2, Motor_Dynamics_2/1, Bus Creator/2
  Throttle To RPM Gain and Cutoff_3/1(Out5) -> Sum/2, Motor_Dynamics_3/1, Bus Creator/3
  Throttle To RPM Gain and Cutoff_4/1(Out5) -> Sum9/2, Motor_Dynamics_4/1, Bus Creator/4
  Motor_Dynamics_1/1 -> Sum3/2, RPM1/1
  Motor_Dynamics_2/1 -> Sum2/2, RPM2/1
  Motor_Dynamics_3/1 -> Sum1/2, RPM3/1
  Motor_Dynamics_4/1 -> Sum4/2, RPM4/1
  Bus Creator/1 -> [B]  "mc and RPM"
  Motor_Dynamics_5/1 -> Sum5/2, RPM5/1
  mc5/1 -> Signal_Saturation_5/1
  Signal_Saturation_5/1 -> Bus Creator/11, Throttle To RPM Gain and Cutoff_5/1(In5)
  Throttle To RPM Gain and Cutoff_5/1(Out5) -> Sum10/2, Motor_Dynamics_5/1, Bus Creator/5
  Motor_Dynamics_6/1 -> Sum6/2, RPM6/1
  mc6/1 -> Signal_Saturation_6/1
  Signal_Saturation_6/1 -> Bus Creator/12, Throttle To RPM Gain and Cutoff_6/1(In5)
  Throttle To RPM Gain and Cutoff_6/1(Out5) -> Sum11/2, Motor_Dynamics_6/1, Bus Creator/6
  Mux/1 -> Demux/1, [RPM_residual]
  Measurement Noise/1 -> Sum1/1
  Sum1/1 -> Sum/1
  Measurement Noise5/1 -> Sum6/1
  Measurement Noise4/1 -> Sum5/1
  Measurement Noise3/1 -> Sum4/1
  Measurement Noise1/1 -> Sum2/1
  Measurement Noise2/1 -> Sum3/1
  Sum2/1 -> Sum8/1
  Sum3/1 -> Sum7/1
  Sum4/1 -> Sum9/1
  Sum5/1 -> Sum10/1
  Sum6/1 -> Sum11/1
  Sum7/1 -> Mux/1
  Sum8/1 -> Mux/2
  Sum/1 -> Mux/3
  Sum9/1 -> Mux/4
  Sum10/1 -> Mux/5
  Sum11/1 -> Mux/6
  Demux/6 -> Scope/6  "R6"
  Demux/5 -> Scope/5  "R5"
  Demux/4 -> Scope/4  "R4"
  Demux/3 -> Scope/3  "R3"
  Demux/2 -> Scope/2  "R2"
  Demux/1 -> Scope/1  "R1"

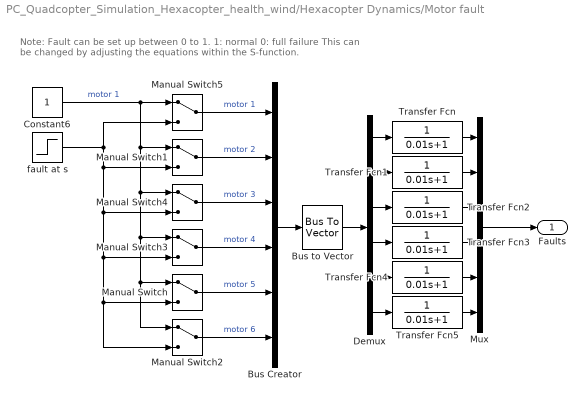
== system PC_Quadcopter_Simulation_Hexacopter_health_wind/Hexacopter Dynamics/Motor fault ==
  note: Note: Fault can be set up between 0 to 1.
      | 1: normal
      | 0: full failure
      | This can be changed by adjusting the equations within the S-function.
  Bus Creator : BusCreator  Inputs=6
  Bus to Vector : BusToVector
  Constant6 : Constant
  Demux : Demux  Outputs=6
  Manual Switch{,1..5} (6 alike) : ManualSwitch
  Mux : Mux  Inputs=6
  Transfer Fcn{,1..5} (6 alike) : TransferFcn  Numerator=1  Denominator=[0.01 1]
  fault at s : Step  Time=85  Before=1  After=0.4  SampleTime=0
  Faults : Outport
  wires:
  Manual Switch1/1 -> Bus Creator/2  "motor 2"
  Manual Switch/1 -> Bus Creator/5  "motor 5"
  Bus Creator/1 -> Bus to Vector/1
  Manual Switch2/1 -> Bus Creator/6  "motor 6"
  Manual Switch3/1 -> Bus Creator/4  "motor 4"
  Demux/1 -> Transfer Fcn/1
  Demux/2 -> Transfer Fcn1/1
  Demux/3 -> Transfer Fcn2/1
  Demux/6 -> Transfer Fcn5/1
  Demux/5 -> Transfer Fcn4/1
  Demux/4 -> Transfer Fcn3/1
  Transfer Fcn/1 -> Mux/1
  Transfer Fcn1/1 -> Mux/2
  Transfer Fcn2/1 -> Mux/3
  Transfer Fcn4/1 -> Mux/5
  Transfer Fcn5/1 -> Mux/6
  Transfer Fcn3/1 -> Mux/4
  Manual Switch4/1 -> Bus Creator/3  "motor 3"
  Constant6/1 -> Manual Switch5/1, Manual Switch2/1, Manual Switch/1, Manual Switch3/1, Manual Switch4/1, Manual Switch1/1  "motor 1"
  Manual Switch5/1 -> Bus Creator/1  "motor 1"
  fault at s/1 -> Manual Switch5/2, Manual Switch2/2, Manual Switch/2, Manual Switch3/2, Manual Switch4/2, Manual Switch1/2
  Bus to Vector/1 -> Demux/1
  Mux/1 -> Faults/1

== system PC_Quadcopter_Simulation_Hexacopter_health_wind/Hexacopter Dynamics/a_x, a_y, a_z ==
  p : Inport
  q : Inport  Port=2
  r : Inport  Port=3
  U : Inport  Port=4
  V : Inport  Port=5
  W : Inport  Port=6
  Phi : Inport  Port=7
  Theta : Inport  Port=8
  Subsystem : Subsystem
  Subsystem1 : Subsystem
  Subsystem2 : Subsystem
  a_x : Outport
  a_y : Outport  Port=2
  a_z : Outport  Port=3
  wires:
  Subsystem/1(a_x) -> a_x/1
  Subsystem1/1(a_y) -> a_y/1
  Subsystem2/1(a_z) -> a_z/1
  q/1 -> Subsystem2/2(q), Subsystem/1(q)
  r/1 -> Subsystem/2(r), Subsystem1/2(r)
  U/1 -> Subsystem2/3(U), Subsystem1/3(U), Subsystem/3(U)
  V/1 -> Subsystem2/4(V), Subsystem/4(V), Subsystem1/4(V)
  W/1 -> Subsystem2/5(W), Subsystem/5(W), Subsystem1/5(W)
  Theta/1 -> Subsystem2/7(Theta), Subsystem1/7(Theta), Subsystem/6(Theta)
  p/1 -> Subsystem2/1(p), Subsystem1/1(p)
  Phi/1 -> Subsystem2/6(Phi), Subsystem1/6(Phi)

== system PC_Quadcopter_Simulation_Hexacopter_health_wind/LESO/Linear Extended-State Observer ==
  y : Inport
  u : Inport  Port=2
  Add3 : Sum  Inputs=+++
  Demux : Demux  Outputs=3
  Integrator : Integrator
  Terminator : Terminator
  theta1 : Gain  Gain=B  Multiplication=Matrix(K*u)
  theta10 : Gain  Gain=L  Multiplication=Matrix(K*u)
  theta2 : Gain  Gain=A-L*C  Multiplication=Matrix(K*u)
  x2_hat : Outport
  x3_hat (F) : Outport  Port=2
  wires:
  theta1/1 -> Add3/2
  theta10/1 -> Add3/1
  y/1 -> theta10/1
  u/1 -> theta1/1
  Add3/1 -> Integrator/1
  theta2/1 -> Add3/3
  Demux/3 -> x3_hat (F)/1
  Demux/2 -> x2_hat/1
  Integrator/1 -> theta2/1, Demux/1
  Demux/1 -> Terminator/1

== system PC_Quadcopter_Simulation_Hexacopter_health_wind/LESO/Linear Extended-State Observer1 ==
  y : Inport
  u : Inport  Port=2
  Add3 : Sum  Commented=on  Inputs=+++
  Demux : Demux  Commented=on  Outputs=3
  Integrator : Integrator  Commented=on
  Terminator : Terminator  Commented=on
  theta1 : Gain  Commented=on  Gain=B  Multiplication=Matrix(K*u)
  theta10 : Gain  Commented=on  Gain=L  Multiplication=Matrix(K*u)
  theta2 : Gain  Commented=on  Gain=A-L*C  Multiplication=Matrix(K*u)
  x2_hat : Outport
  x3_hat (F) : Outport  Port=2
  wires:
  Demux/1 -> Terminator/1
  Integrator/1 -> Demux/1, theta2/1
  Demux/2 -> x2_hat/1
  Demux/3 -> x3_hat (F)/1
  theta2/1 -> Add3/3
  Add3/1 -> Integrator/1
  u/1 -> theta1/1
  y/1 -> theta10/1
  theta10/1 -> Add3/1
  theta1/1 -> Add3/2

== system PC_Quadcopter_Simulation_Hexacopter_health_wind/LESO/Linear Extended-State Observer2 ==
  y : Inport
  u : Inport  Port=2
  Add3 : Sum  Inputs=+++
  Demux : Demux  Outputs=3
  Integrator : Integrator
  Terminator : Terminator
  theta1 : Gain  Gain=B  Multiplication=Matrix(K*u)
  theta10 : Gain  Gain=L  Multiplication=Matrix(K*u)
  theta2 : Gain  Gain=A-L*C  Multiplication=Matrix(K*u)
  x2_hat : Outport
  x3_hat (F) : Outport  Port=2
  wires:
  theta1/1 -> Add3/2
  theta10/1 -> Add3/1
  y/1 -> theta10/1
  u/1 -> theta1/1
  Add3/1 -> Integrator/1
  theta2/1 -> Add3/3
  Demux/3 -> x3_hat (F)/1
  Demux/2 -> x2_hat/1
  Integrator/1 -> theta2/1, Demux/1
  Demux/1 -> Terminator/1

== system PC_Quadcopter_Simulation_Hexacopter_health_wind/Position Controller/Altitude (Z) Control ==
  note: Improve to use rotation matrix and euler angles...
      | maybe with saturation?
  note: ez
  Desired Z : Inport
  Bus Selector : BusSelector  OutputSignals=Alt_Cmd
  Gravity Offset (Level Flight) : Constant  Value=GOffset
  Integrator Limited : Integrator  LimitOutput=on  UpperSaturationLimit=USat  LowerSaturationLimit=LSat
  Kiz : Gain  Gain=Kiz
  Kpz : Gain  Gain=Kpz
  Sum : Sum  Inputs=|+|
  Sum2 : Sum  Inputs=+++
  Alt. (Z) Correction : Outport
  wires:
  Gravity Offset (Level Flight)/1 -> Sum2/1
  Desired Z/1 -> Bus Selector/1
  Sum2/1 -> Alt. (Z) Correction/1
  Kpz/1 -> Sum2/2  "P Corr"
  Sum/1 -> Integrator Limited/1, Kpz/1  "Error"
  Kiz/1 -> Sum2/3  "I Corr"
  Integrator Limited/1 -> Kiz/1
  Bus Selector/1 -> Sum/1  "<Alt_Cmd>"

== system PC_Quadcopter_Simulation_Hexacopter_health_wind/Position Controller/Altitude (Z) Control1 ==
  note: ez
  note: Improve to use rotation matrix and euler angles...
      | maybe with saturation?
  Desired Z : Inport
  Bus Selector : BusSelector  OutputSignals=Alt_Cmd
  Gravity Offset (Level Flight) : Constant  Value=GOffset
  Integrator Limited : Integrator  LimitOutput=on  UpperSaturationLimit=USat  LowerSaturationLimit=LSat
  Kiz : Gain  Gain=Kiz
  Kpz : Gain  Gain=Kpz
  Sum : Sum  Inputs=|+|
  Sum2 : Sum  Inputs=+++
  Alt. (Z) Correction : Outport
  wires:
  Bus Selector/1 -> Sum/1  "<Alt_Cmd>"
  Integrator Limited/1 -> Kiz/1
  Kiz/1 -> Sum2/3  "I Corr"
  Sum/1 -> Kpz/1, Integrator Limited/1  "Error"
  Kpz/1 -> Sum2/2  "P Corr"
  Sum2/1 -> Alt. (Z) Correction/1
  Desired Z/1 -> Bus Selector/1
  Gravity Offset (Level Flight)/1 -> Sum2/1

== system PC_Quadcopter_Simulation_Hexacopter_health_wind/Position Controller/Error Rotations ==
  X_cmd : Inport
  Y_cmd : Inport  Port=2
  X : Inport  Port=3
  Y : Inport  Port=4
  Psi : Inport  Port=5
  Product{,1..3} (4 alike) : Product
  Sum : Sum  Inputs=|+-
  Sum1 : Sum  Inputs=|+-
  Sum2 : Sum  Inputs=|++
  Sum4 : Sum  Inputs=|+-
  Trigonometric Functions : Trigonometry  Operator=sincos
  X Error in body Frame : Outport
  Y Error in Body Frame : Outport  Port=2
  wires:
  Sum4/1 -> Y Error in Body Frame/1  "Yerr*cos(psi)-Xerr*sin(psi)"
  Product3/1 -> Sum4/2  "Xerr*sin(psi)"
  Sum1/1 -> Product2/1, Product1/1  "Y Error"
  Trigonometric Functions/1 -> Product2/2, Product3/2  "sin(psi)"
  Sum2/1 -> X Error in body Frame/1  "Xerr*cos(psi)+Yerr*sin(psi)"
  Y_cmd/1 -> Sum1/1
  X_cmd/1 -> Sum/1
  X/1 -> Sum/2
  Y/1 -> Sum1/2
  Sum/1 -> Product3/1, Product/1  "X Error"
  Trigonometric Functions/2 -> Product/2, Product1/2  "cos(psi)"
  Product/1 -> Sum2/1  "Xerr*cos(psi)"
  Product2/1 -> Sum2/2  "Yerr*sin(psi)"
  Product1/1 -> Sum4/1  "Yerr*cos(psi)"
  Psi/1 -> Trigonometric Functions/1

== system PC_Quadcopter_Simulation_Hexacopter_health_wind/Position Controller/Error Rotations1 ==
  X_cmd : Inport
  Y_cmd : Inport  Port=2
  Constant : Constant  Value=0
  Product{,1..3} (4 alike) : Product
  Sum2 : Sum  Inputs=|++
  Sum4 : Sum  Inputs=|+-
  Trigonometric Functions : Trigonometry  Operator=sincos
  X Error in body Frame : Outport
  Y Error in Body Frame : Outport  Port=2
  wires:
  Constant/1 -> Trigonometric Functions/1
  Product1/1 -> Sum4/1  "Yerr*cos(psi)"
  Product2/1 -> Sum2/2  "Yerr*sin(psi)"
  Product/1 -> Sum2/1  "Xerr*cos(psi)"
  Trigonometric Functions/2 -> Product1/2, Product/2  "cos(psi)"
  X_cmd/1 -> Product/1, Product3/1  "X Error"
  Sum2/1 -> X Error in body Frame/1  "Xerr*cos(psi)+Yerr*sin(psi)"
  Trigonometric Functions/1 -> Product3/2, Product2/2  "sin(psi)"
  Y_cmd/1 -> Product1/1, Product2/1  "Y Error"
  Product3/1 -> Sum4/2  "Xerr*sin(psi)"
  Sum4/1 -> Y Error in Body Frame/1  "Yerr*cos(psi)-Xerr*sin(psi)"

== system PC_Quadcopter_Simulation_Hexacopter_health_wind/Position Controller/Error Rotations2 ==
  X_cmd : Inport
  Y_cmd : Inport  Port=2
  X : Inport  Port=3
  Y : Inport  Port=4
  Psi : Inport  Port=5
  Product{,1..3} (4 alike) : Product
  Sum : Sum  Inputs=|+-
  Sum1 : Sum  Inputs=|+-
  Sum2 : Sum  Inputs=|++
  Sum4 : Sum  Inputs=|+-
  Trigonometric Functions : Trigonometry  Operator=sincos
  X Error in body Frame : Outport
  Y Error in Body Frame : Outport  Port=2
  wires:
  Psi/1 -> Trigonometric Functions/1
  Product1/1 -> Sum4/1  "Yerr*cos(psi)"
  Product2/1 -> Sum2/2  "Yerr*sin(psi)"
  Product/1 -> Sum2/1  "Xerr*cos(psi)"
  Trigonometric Functions/2 -> Product1/2, Product/2  "cos(psi)"
  Sum/1 -> Product/1, Product3/1  "X Error"
  Y/1 -> Sum1/2
  X/1 -> Sum/2
  X_cmd/1 -> Sum/1
  Y_cmd/1 -> Sum1/1
  Sum2/1 -> X Error in body Frame/1  "Xerr*cos(psi)+Yerr*sin(psi)"
  Trigonometric Functions/1 -> Product3/2, Product2/2  "sin(psi)"
  Sum1/1 -> Product1/1, Product2/1  "Y Error"
  Product3/1 -> Sum4/2  "Xerr*sin(psi)"
  Sum4/1 -> Y Error in Body Frame/1  "Yerr*cos(psi)-Xerr*sin(psi)"

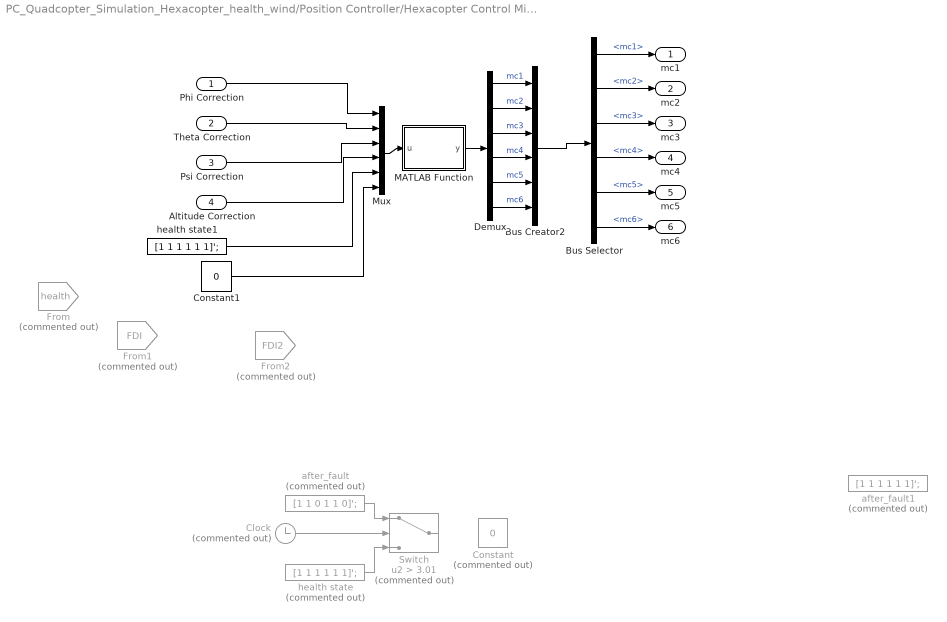
== system PC_Quadcopter_Simulation_Hexacopter_health_wind/Position Controller/Hexacopter Control Mixing ==
  Phi Correction : Inport
  Theta Correction : Inport  Port=2
  Psi Correction : Inport  Port=3
  Altitude Correction : Inport  Port=4
  Bus Creator2 : BusCreator  Inputs=6
  Bus Selector : BusSelector  OutputSignals=mc1,mc2,mc3,mc4,mc5,mc6
  Clock : Clock  Commented=on
  Constant : Constant  Commented=on  Value=0
  Constant1 : Constant  Value=0
  Demux : Demux  Outputs=6
  From : From  Commented=on  GotoTag=health  TagVisibility=global
  From1 : From  Commented=on  GotoTag=FDI  TagVisibility=global
  From2 : From  Commented=on  GotoTag=FDI2  TagVisibility=global
  MATLAB Function : MATLAB Function  TreatAsAtomicUnit=on
  Mux : Mux  Inputs=6
  Switch : Switch  Commented=on  Criteria=u2 > Threshold  Threshold=3.01  SaturateOnIntegerOverflow=off  InputSameDT=off
  after_fault : Constant  Commented=on  Value=[1 1 0 1 1 0]';
  after_fault1 : Constant  Commented=on  Value=[1 1 1 1 1 1]';
  health state : Constant  Commented=on  Value=[1 1 1 1 1 1]';
  health state1 : Constant  Value=[1 1 1 1 1 1]';
  mc1 : Outport
  mc2 : Outport  Port=2
  mc3 : Outport  Port=3
  mc4 : Outport  Port=4
  mc5 : Outport  Port=5
  mc6 : Outport  Port=6
  wires:
  Phi Correction/1 -> Mux/1
  Theta Correction/1 -> Mux/2
  Psi Correction/1 -> Mux/3
  Altitude Correction/1 -> Mux/4
  Bus Selector/1 -> mc1/1  "<mc1>"
  Bus Selector/2 -> mc2/1  "<mc2>"
  Bus Selector/3 -> mc3/1  "<mc3>"
  Bus Selector/4 -> mc4/1  "<mc4>"
  Bus Selector/5 -> mc5/1  "<mc5>"
  Bus Selector/6 -> mc6/1  "<mc6>"
  Mux/1 -> MATLAB Function/1(u)
  MATLAB Function/1(y) -> Demux/1
  Demux/6 -> Bus Creator2/6  "mc6"
  Demux/3 -> Bus Creator2/3  "mc3"
  Demux/4 -> Bus Creator2/4  "mc4"
  Demux/1 -> Bus Creator2/1  "mc1"
  Demux/5 -> Bus Creator2/5  "mc5"
  Demux/2 -> Bus Creator2/2  "mc2"
  Bus Creator2/1 -> Bus Selector/1
  Constant1/1 -> Mux/6
  health state1/1 -> Mux/5
  health state/1 -> Switch/3
  after_fault/1 -> Switch/1
  Clock/1 -> Switch/2

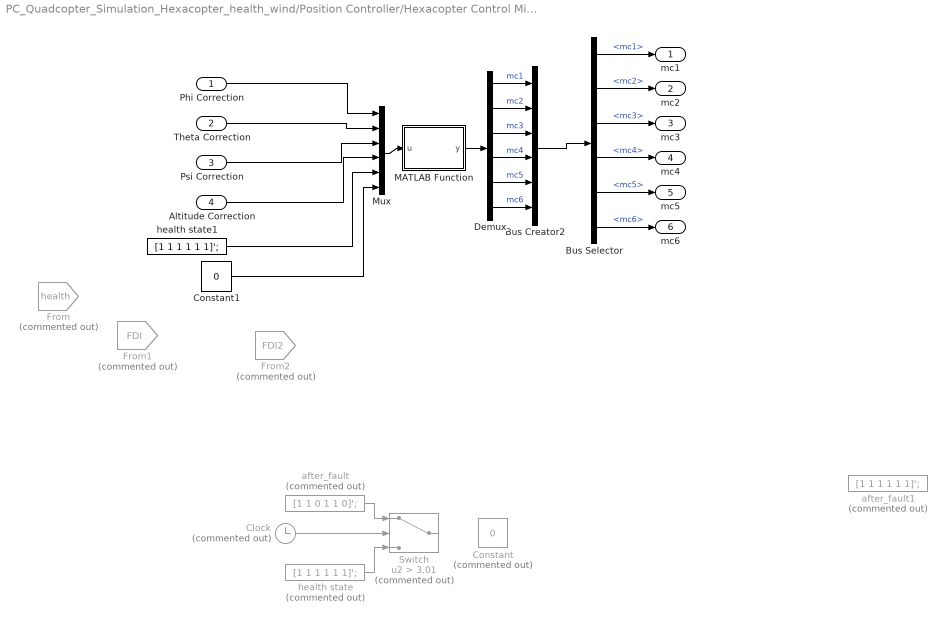
== system PC_Quadcopter_Simulation_Hexacopter_health_wind/Position Controller/Hexacopter Control Mixing1 ==
  Phi Correction : Inport
  Theta Correction : Inport  Port=2
  Psi Correction : Inport  Port=3
  Altitude Correction : Inport  Port=4
  Bus Creator2 : BusCreator  Inputs=6
  Bus Selector : BusSelector  OutputSignals=mc1,mc2,mc3,mc4,mc5,mc6
  Clock : Clock  Commented=on
  Constant : Constant  Commented=on  Value=0
  Constant1 : Constant  Value=0
  Demux : Demux  Outputs=6
  From : From  Commented=on  GotoTag=health  TagVisibility=global
  From1 : From  Commented=on  GotoTag=FDI  TagVisibility=global
  From2 : From  Commented=on  GotoTag=FDI2  TagVisibility=global
  MATLAB Function : MATLAB Function  TreatAsAtomicUnit=on
  Mux : Mux  Inputs=6
  Switch : Switch  Commented=on  Criteria=u2 > Threshold  Threshold=3.01  SaturateOnIntegerOverflow=off  InputSameDT=off
  after_fault : Constant  Commented=on  Value=[1 1 0 1 1 0]';
  after_fault1 : Constant  Commented=on  Value=[1 1 1 1 1 1]';
  health state : Constant  Commented=on  Value=[1 1 1 1 1 1]';
  health state1 : Constant  Value=[1 1 1 1 1 1]';
  mc1 : Outport
  mc2 : Outport  Port=2
  mc3 : Outport  Port=3
  mc4 : Outport  Port=4
  mc5 : Outport  Port=5
  mc6 : Outport  Port=6
  wires:
  Clock/1 -> Switch/2
  after_fault/1 -> Switch/1
  health state/1 -> Switch/3
  health state1/1 -> Mux/5
  Constant1/1 -> Mux/6
  Bus Creator2/1 -> Bus Selector/1
  Demux/2 -> Bus Creator2/2  "mc2"
  Demux/5 -> Bus Creator2/5  "mc5"
  Demux/1 -> Bus Creator2/1  "mc1"
  Demux/4 -> Bus Creator2/4  "mc4"
  Demux/3 -> Bus Creator2/3  "mc3"
  Demux/6 -> Bus Creator2/6  "mc6"
  MATLAB Function/1(y) -> Demux/1
  Mux/1 -> MATLAB Function/1(u)
  Bus Selector/6 -> mc6/1  "<mc6>"
  Bus Selector/5 -> mc5/1  "<mc5>"
  Bus Selector/4 -> mc4/1  "<mc4>"
  Bus Selector/3 -> mc3/1  "<mc3>"
  Bus Selector/2 -> mc2/1  "<mc2>"
  Bus Selector/1 -> mc1/1  "<mc1>"
  Altitude Correction/1 -> Mux/4
  Psi Correction/1 -> Mux/3
  Theta Correction/1 -> Mux/2
  Phi Correction/1 -> Mux/1

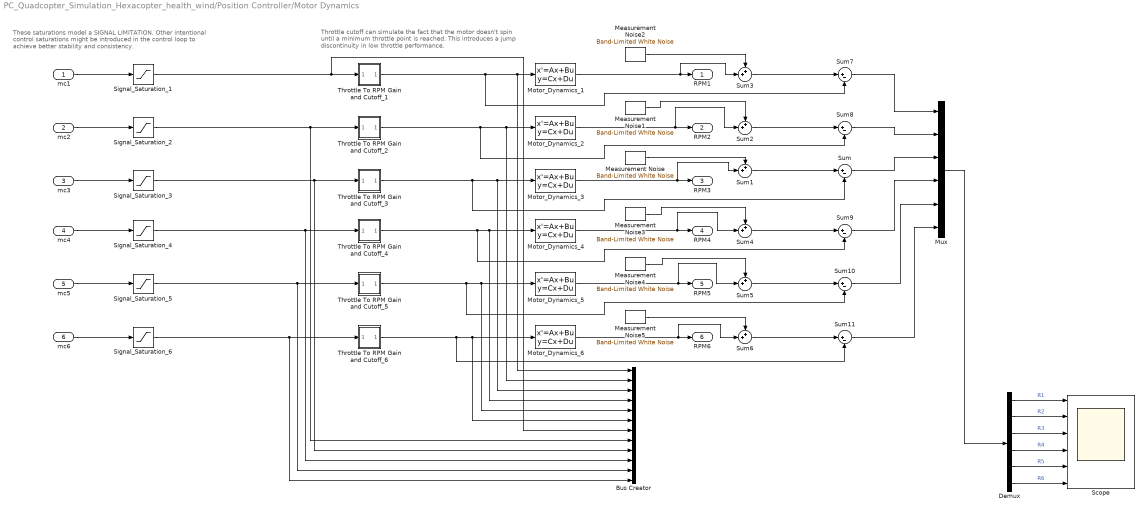
== system PC_Quadcopter_Simulation_Hexacopter_health_wind/Position Controller/Motor Dynamics ==
  note: Throttle cutoff can simulate the fact that the motor doesn't
      | spin until a minimum throttle point is reached. This introduces
      | a jump discontinuity in low throttle performance.
  note: These saturations model a SIGNAL LIMITATION.
      | Other intentional control saturations might be introduced in the
      | control loop to achieve better stability and consistency.
  mc1 : Inport
  mc2 : Inport  Port=2
  mc3 : Inport  Port=3
  mc4 : Inport  Port=4
  mc5 : Inport  Port=5
  mc6 : Inport  Port=6
  Bus Creator : BusCreator  Inputs=12
  Demux : Demux  Outputs=6
  Measurement Noise{,1..5} (6 alike) : simulink/Sources/Band-Limited White Noise  Cov=10^2  Ts=0.02  seed=[23342]
  Motor_Dynamics_1 : StateSpace  A=-1/quadModel.T  C=1/quadModel.T  D=0  InitialCondition=IC.w1*quadModel.T
  Motor_Dynamics_2 : StateSpace  A=-1/quadModel.T  C=1/quadModel.T  D=0  InitialCondition=IC.w2*quadModel.T
  Motor_Dynamics_3 : StateSpace  A=-1/quadModel.T  C=1/quadModel.T  D=0  InitialCondition=IC.w3*quadModel.T
  Motor_Dynamics_4 : StateSpace  A=-1/quadModel.T  C=1/quadModel.T  D=0  InitialCondition=IC.w4*quadModel.T
  Motor_Dynamics_5 : StateSpace  A=-1/quadModel.T  C=1/quadModel.T  D=0  InitialCondition=IC.w4*quadModel.T
  Motor_Dynamics_6 : StateSpace  A=-1/quadModel.T  C=1/quadModel.T  D=0  InitialCondition=IC.w4*quadModel.T
  Mux : Mux  Inputs=6
  Scope : Scope  NumInputPorts=6
  Signal_Saturation_{1..6} (6 alike) : Saturate  UpperLimit=100  LowerLimit=0
  Sum{,7..11} (6 alike) : Sum  Inputs=|+-
  Sum{1..6} (6 alike) : Sum  Inputs=++|
  Throttle To RPM Gain and Cutoff_1 : Subsystem
  Throttle To RPM Gain and Cutoff_2 : Subsystem
  Throttle To RPM Gain and Cutoff_3 : Subsystem
  Throttle To RPM Gain and Cutoff_4 : Subsystem
  Throttle To RPM Gain and Cutoff_5 : Subsystem
  Throttle To RPM Gain and Cutoff_6 : Subsystem
  RPM1 : Outport
  RPM2 : Outport  Port=2
  RPM3 : Outport  Port=3
  RPM4 : Outport  Port=4
  RPM5 : Outport  Port=5
  RPM6 : Outport  Port=6
  wires:
  mc1/1 -> Signal_Saturation_1/1
  mc4/1 -> Signal_Saturation_4/1
  mc2/1 -> Signal_Saturation_2/1
  mc3/1 -> Signal_Saturation_3/1
  Signal_Saturation_1/1 -> Bus Creator/7, Throttle To RPM Gain and Cutoff_1/1(In5)
  Signal_Saturation_2/1 -> Throttle To RPM Gain and Cutoff_2/1(In5), Bus Creator/8
  Signal_Saturation_3/1 -> Bus Creator/9, Throttle To RPM Gain and Cutoff_3/1(In5)
  Signal_Saturation_4/1 -> Bus Creator/10, Throttle To RPM Gain and Cutoff_4/1(In5)
  Throttle To RPM Gain and Cutoff_1/1(Out5) -> Sum7/2, Bus Creator/1, Motor_Dynamics_1/1
  Throttle To RPM Gain and Cutoff_2/1(Out5) -> Sum8/2, Motor_Dynamics_2/1, Bus Creator/2
  Throttle To RPM Gain and Cutoff_3/1(Out5) -> Sum/2, Motor_Dynamics_3/1, Bus Creator/3
  Throttle To RPM Gain and Cutoff_4/1(Out5) -> Sum9/2, Motor_Dynamics_4/1, Bus Creator/4
  Motor_Dynamics_1/1 -> Sum3/2, RPM1/1
  Motor_Dynamics_2/1 -> Sum2/2, RPM2/1
  Motor_Dynamics_3/1 -> Sum1/2, RPM3/1
  Motor_Dynamics_4/1 -> Sum4/2, RPM4/1
  Motor_Dynamics_5/1 -> Sum5/2, RPM5/1
  mc5/1 -> Signal_Saturation_5/1
  Signal_Saturation_5/1 -> Bus Creator/11, Throttle To RPM Gain and Cutoff_5/1(In5)
  Throttle To RPM Gain and Cutoff_5/1(Out5) -> Sum10/2, Motor_Dynamics_5/1, Bus Creator/5
  Motor_Dynamics_6/1 -> Sum6/2, RPM6/1
  mc6/1 -> Signal_Saturation_6/1
  Signal_Saturation_6/1 -> Bus Creator/12, Throttle To RPM Gain and Cutoff_6/1(In5)
  Throttle To RPM Gain and Cutoff_6/1(Out5) -> Sum11/2, Motor_Dynamics_6/1, Bus Creator/6
  Mux/1 -> Demux/1
  Measurement Noise/1 -> Sum1/1
  Sum1/1 -> Sum/1
  Measurement Noise5/1 -> Sum6/1
  Measurement Noise4/1 -> Sum5/1
  Measurement Noise3/1 -> Sum4/1
  Measurement Noise1/1 -> Sum2/1
  Measurement Noise2/1 -> Sum3/1
  Sum2/1 -> Sum8/1
  Sum3/1 -> Sum7/1
  Sum4/1 -> Sum9/1
  Sum5/1 -> Sum10/1
  Sum6/1 -> Sum11/1
  Sum7/1 -> Mux/1
  Sum8/1 -> Mux/2
  Sum/1 -> Mux/3
  Sum9/1 -> Mux/4
  Sum10/1 -> Mux/5
  Sum11/1 -> Mux/6
  Demux/6 -> Scope/6  "R6"
  Demux/5 -> Scope/5  "R5"
  Demux/4 -> Scope/4  "R4"
  Demux/3 -> Scope/3  "R3"
  Demux/2 -> Scope/2  "R2"
  Demux/1 -> Scope/1  "R1"
